simulink model "L1E1a3"  (R2020b)
settings: Solver=VariableStepAuto  StartTime=0.0  StopTime=10.0  RelTol=1e-3
settings Model: Creator=Vedant Nath  LastModifiedBy=Vedant Nath

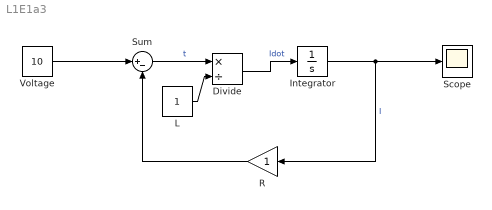
== system L1E1a3 ==
  Divide : Product  Inputs=*/
  Integrator : Integrator
  L : Constant
  R : Gain
  Scope : Scope
  Sum : Sum  Inputs=|+-
  Voltage : Constant  Value=10
  wires:
  Voltage/1 -> Sum/1
  Integrator/1 -> Scope/1, R/1  "I"
  R/1 -> Sum/2
  Sum/1 -> Divide/1  "t"
  Divide/1 -> Integrator/1  "Idot"
  L/1 -> Divide/2
